simulink model "demoqp_e"  (R2020b)
settings: Solver=VariableStepAuto  StartTime=0.0  StopTime=10.0  RelTol=1e-3
settings Model: Creator=abhis  LastModifiedBy=abhis

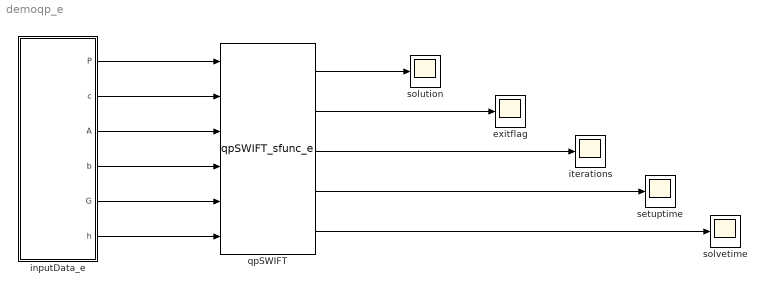
== system demoqp_e ==
  exitflag : Scope
  inputData_e : MATLAB Function  TreatAsAtomicUnit=on
  iterations : Scope
  qpSWIFT : S-Function  FunctionName=qpSWIFT_sfunc_e  SFunctionDeploymentMode=off  EnableBusSupport=off
  setuptime : Scope
  solution : Scope
  solvetime : Scope
  wires:
  inputData_e/1(P) -> qpSWIFT/1
  inputData_e/2(c) -> qpSWIFT/2
  inputData_e/3(A) -> qpSWIFT/3
  inputData_e/4(b) -> qpSWIFT/4
  inputData_e/5(G) -> qpSWIFT/5
  inputData_e/6(h) -> qpSWIFT/6
  qpSWIFT/1 -> solution/1
  qpSWIFT/2 -> exitflag/1
  qpSWIFT/3 -> iterations/1
  qpSWIFT/4 -> setuptime/1
  qpSWIFT/5 -> solvetime/1

== matlab function demoqp_e/inputData_e ==
  data: P output; c output; A output; b output; G output; h output
function [P,c,A,b,G,h] = fcn()


in_P = [5 1 0; 1 2 1; 0 1 4];
c = [1; 2; 1];


%%%% Equality Constraints
in_A = [1 -2 1];
b = 3;


%%%% Inequality Constraints
in_G = [-4 -4 0; 0 0 -1];
h = [-1; -1];



%%%% Matrices are ordered in column major format
P = in_P(:);
A = in_A(:);
G = in_G(:);


end
